simulink model "Ex2_SysIdentification"  (R2023b)
settings: Solver=FixedStepDiscrete  StartTime=0.0  StopTime=inf  FixedStep=0.1  RelTol=1e-3  EnableMultiTasking=on
libraries: arduinolib x1, arduinosensorlib x1
settings Model: ExtModeTrigDuration=2  Creator=Alejandro  LastModifiedBy=Alejandro
settings OptimizationCC: EnhancedBackFolding=on  PassReuseOutputArgsAs=Individual arguments  ZeroExternalMemoryAtStartup=off  ZeroInternalMemoryAtStartup=off  MaxStackSize=64  OptimizeBlockOrder=speed  DifferentSizesBufferReuse=on  OptimizationCustomize=off  EfficientTunableParamExpr=on
settings DebuggingCC: ParameterTunabilityLossMsg=error
settings HardwareCC: ProdBitPerInt=16  ProdBitPerPointer=16  ProdBitPerSizeT=16  ProdBitPerPtrDiffT=16  ProdLargestAtomicFloat=None  ProdWordSize=8  ProdHWDeviceType=Atmel->AVR
settings SFSimCC: MATLABDynamicMemAlloc=off
settings RTWCC: Description=Embedded Coder  SystemTargetFile=ert.tlc  HardwareBoard=Arduino Uno  TemplateMakefile=ert_default_tmf  Toolchain=Arduino AVR  BuildConfiguration=Faster Runs
settings CodeAppCC: ForceParamTrailComments=on  IgnoreCustomStorageClasses=off  OperatorAnnotations=on  SimulinkDataObjDesc=on  SFDataObjDesc=on  InsertBlockDesc=on
settings ERTTargetCC: SupportContinuousTime=on  SupportVariableSizeSignals=on  ExtModeTransport=3  ExtModeStaticAlloc=on  ExtModeAutomaticAllocSize=off  ExtModeStaticAllocSize=250  ExtModeMexFile=ext_xcp  ExtModeIntrfLevel=Level2 - Open

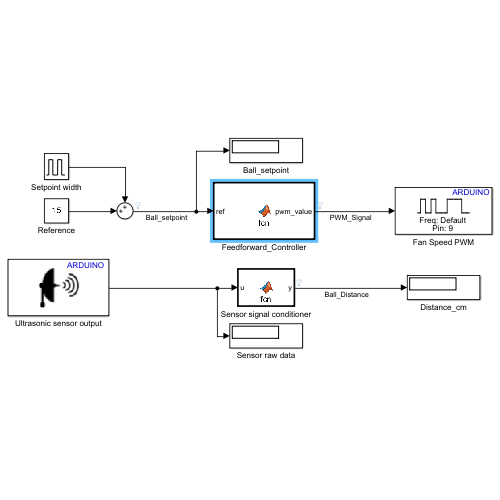
[thumbnail: Simulink's stored preview of the top-level diagram]
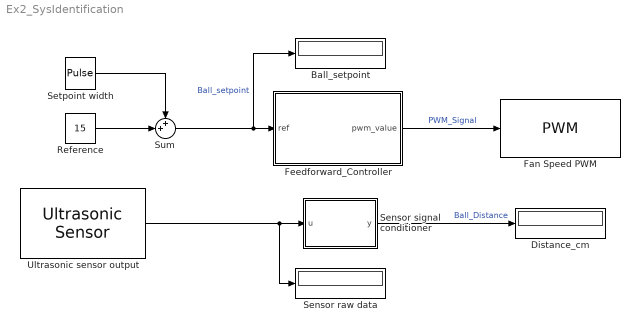
== system Ex2_SysIdentification ==
  Ball_setpoint : Display
  Distance_cm : Display
  Fan Speed PWM : arduinolib/PWM  pinNumber=9  frequencyType=Default  desiredFrequency=490.2  achievableFrequency=490.2
  Feedforward_Controller : MATLAB Function  TreatAsAtomicUnit=on
  Reference : Constant  Value=15
  Sensor raw data : Display
  Sensor signal conditioner : MATLAB Function  TreatAsAtomicUnit=on
  Setpoint width : DiscretePulseGenerator  PulseType=Time based  Amplitude=10  Period=20  PulseWidth=50
  Sum : Sum  Inputs=++|
  Ultrasonic sensor output : arduinosensorlib/Ultrasonic Sensor  NumSignalPins=2  TrigPin=12  EchoPin=11  SignalPin=3  SampleTime_=0.1  blockPlatform=ARDUINO
  wires:
  Ultrasonic sensor output/1 -> Sensor signal conditioner/1(u), Sensor raw data/1
  Sensor signal conditioner/1(y) -> Distance_cm/1  "Ball_Distance"
  Sum/1 -> Ball_setpoint/1, Feedforward_Controller/1(ref)  "Ball_setpoint"
  Feedforward_Controller/1(pwm_value) -> Fan Speed PWM/1  "PWM_Signal"
  Setpoint width/1 -> Sum/1
  Reference/1 -> Sum/2

== matlab function Ex2_SysIdentification/Sensor signal conditioner ==
  data: u input; y output
function y = fcn(u)

MAX_DIST = 30;

y=MAX_DIST-(u*100);

== matlab function Ex2_SysIdentification/Feedforward_Controller ==
  data: pwm_value output; ref input
function pwm_value = fcn(ref)

% Values for the lineal regression obtained in P5
a=0.2678;
b=-19.218;

% Compute the value for the PWM signal with lineal regression
pwm_value=a*ref+b;
